simulink model "tp4_partie4"  (R2016a)
settings: Solver=VariableStepAuto  StartTime=0.0  StopTime=10.0  RelTol=1e-3
values from neighbouring files (symbols this model uses):
  K = [100;10]    [init.m]    (also in init_TP2_controle.m = [20;10]; init_tp3.m = [20 10]; matrices_init_tp4_partie3_4.m = place(A,-B,V))
  L = H/2    (= 0.072)    [matrices_init_tp4_partie3_4.m]
undefined symbols (not defined in the file or in its folder): DiscIntNeverNeededParam
libraries: simulink x2
settings Model: Creator=plarato  LastModifiedBy=plarato

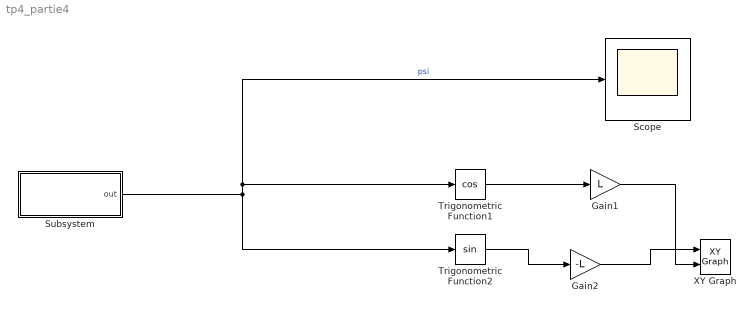
== system tp4_partie4 ==
  Gain1 : Gain  Gain=L
  Gain2 : Gain  Gain=-L
  Scope : Scope
  Subsystem : Subsystem
  Trigonometric Function1 : Trigonometry  Operator=cos
  Trigonometric Function2 : Trigonometry
  XY Graph : simulink/Sinks/XY Graph  xmin=-L  xmax=L  ymin=-L  ymax=L  st=-1
  wires:
  Trigonometric Function1/1 -> Gain1/1
  Trigonometric Function2/1 -> Gain2/1
  Gain2/1 -> XY Graph/1
  Gain1/1 -> XY Graph/2
  Subsystem/1("out ") -> Trigonometric Function2/1, Scope/1, Trigonometric Function1/1  "psi"

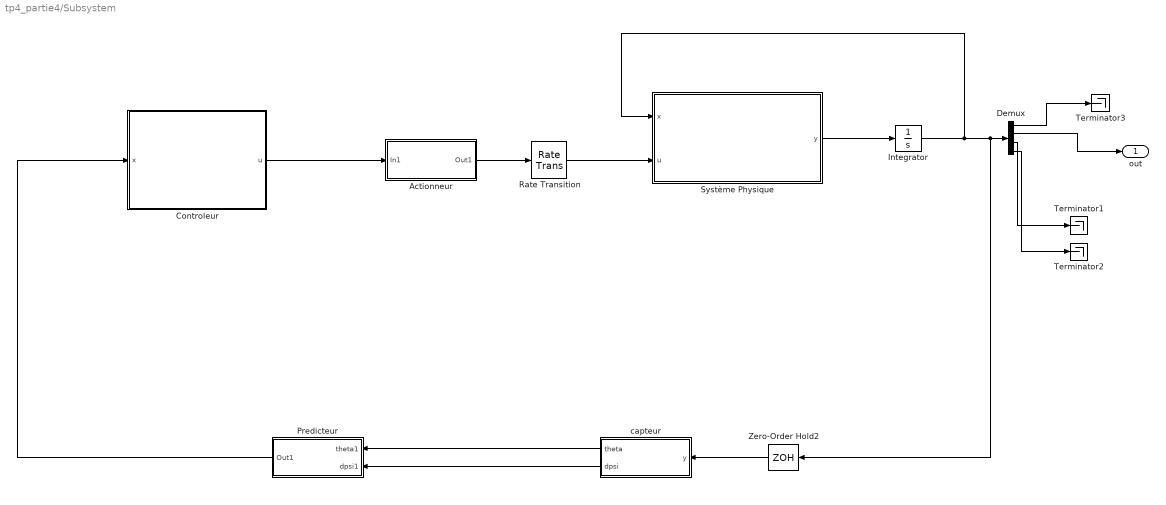
== system tp4_partie4/Subsystem ==
  Actionneur : Subsystem
  Controleur : Subsystem
  Demux : Demux
  Integrator : Integrator  InitialCondition=[pi/4 pi/3 0 0]
  Predicteur : Subsystem
  Rate Transition : RateTransition  OutPortSampleTime=0.002
  "Système Physique " : Subsystem
  Terminator1 : Terminator
  Terminator2 : Terminator
  Terminator3 : Terminator
  Zero-Order Hold2 : ZeroOrderHold  SampleTime=0.002
  "capteur " : Subsystem
  "out " : Outport
  wires:
  Controleur/1(u) -> Actionneur/1(In1)
  Actionneur/1(Out1) -> Rate Transition/1
  Integrator/1 -> "Système Physique "/1(x), Zero-Order Hold2/1, Demux/1
  Predicteur/1(Out1) -> Controleur/1(x)
  "Système Physique "/1("y ") -> Integrator/1
  Demux/3 -> Terminator1/1
  Demux/4 -> Terminator2/1
  Rate Transition/1 -> "Système Physique "/2(u)
  "capteur "/1("theta ") -> Predicteur/1(theta1)
  "capteur "/2(dpsi) -> Predicteur/2("dpsi1 ")
  Zero-Order Hold2/1 -> "capteur "/1(y)
  Demux/2 -> "out "/1
  Demux/1 -> Terminator3/1

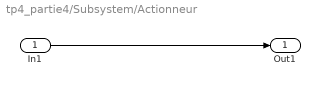
== system tp4_partie4/Subsystem/Actionneur ==
  In1 : Inport
  Out1 : Outport
  wires:
  In1/1 -> Out1/1

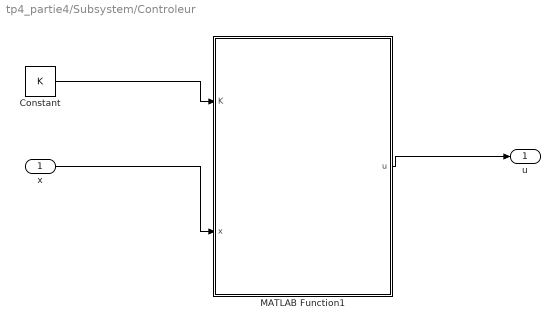
== system tp4_partie4/Subsystem/Controleur ==
  x : Inport
  Constant : Constant  Value=K
  MATLAB Function1 : MATLAB Function  TreatAsAtomicUnit=on
  u : Outport
  wires:
  MATLAB Function1/1(u) -> u/1
  x/1 -> MATLAB Function1/2(x)
  Constant/1 -> MATLAB Function1/1(K)

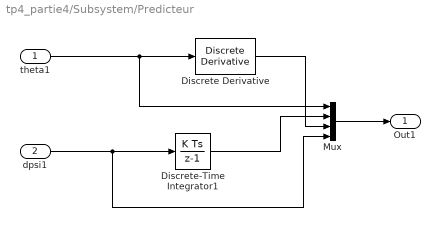
== system tp4_partie4/Subsystem/Predicteur ==
  theta1 : Inport  PortDimensions=1
  "dpsi1 " : Inport  Port=2  PortDimensions=1
  Discrete Derivative : simulink/Discrete/Discrete Derivative  gainval=1.0  ICPrevScaledInput=pi/4  OutMin=[]  OutMax=[]  OutDataType=fixdt(1, 16)  OutScaling=2^-10  DoSatur=off
  Discrete-Time Integrator1 : DiscreteIntegrator  InitialConditionSetting=State (most efficient)  SampleTime=-1  ICPrevOutput=DiscIntNeverNeededParam  ICPrevScaledInput=DiscIntNeverNeededParam
  Mux : Mux
  Out1 : Outport  PortDimensions=4
  wires:
  theta1/1 -> Mux/1, Discrete Derivative/1
  Mux/1 -> Out1/1
  Discrete-Time Integrator1/1 -> Mux/2
  "dpsi1 "/1 -> Mux/4, Discrete-Time Integrator1/1
  Discrete Derivative/1 -> Mux/3

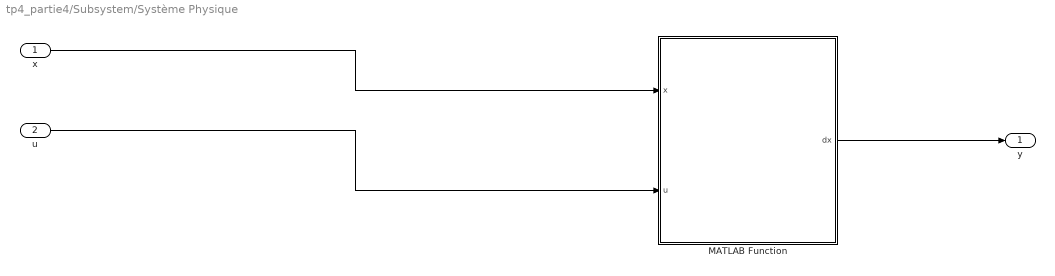
== system tp4_partie4/Subsystem/Système Physique  ==
  x : Inport
  u : Inport  Port=2
  MATLAB Function : MATLAB Function  TreatAsAtomicUnit=on
  "y " : Outport
  wires:
  MATLAB Function/1(dx) -> "y "/1
  u/1 -> MATLAB Function/2(u)
  x/1 -> MATLAB Function/1(x)

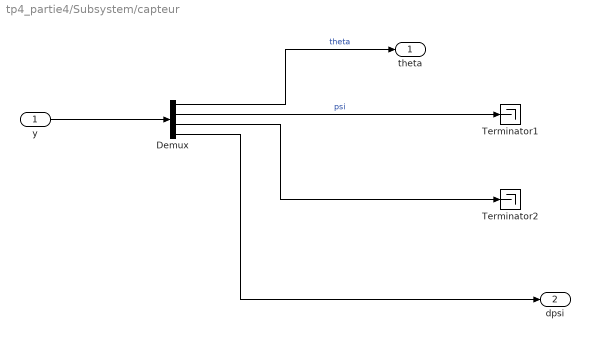
== system tp4_partie4/Subsystem/capteur  ==
  y : Inport  PortDimensions=4
  Demux : Demux
  Terminator1 : Terminator
  Terminator2 : Terminator
  "theta " : Outport  PortDimensions=1
  dpsi : Outport  Port=2  PortDimensions=1
  wires:
  Demux/1 -> "theta "/1  "theta"
  y/1 -> Demux/1
  Demux/3 -> Terminator2/1
  Demux/2 -> Terminator1/1  "psi"
  Demux/4 -> dpsi/1

== matlab function tp4_partie4/Subsystem/Controleur/MATLAB Function1 ==
  data: K input; x input; u output
%Controleur
function u = fcn(K, x)
%#codegen
ue=0;
%K=[20;10];
%K = [0.67; 19.9053; 1.0747; 1.9614];


xe = [0;0;0;0];

u = ue + K'*(x - xe);

== matlab function tp4_partie4/Subsystem/Système Physique /MATLAB Function ==
  data: x input; dx output; u input
function dx   = fonction( x, u)
%   Dynamic equations of motion of the segway on an axis.
%   Inputs: - x = [theta psi dtheta dpsi]
%               theta: average angle of the wheels      [rad]
%               psi: body pitch angle                   [rad]
%               dtheta: average velocity of the wheels  [rad/s]
%               dpsi: body pitch velocity               [rad/s]
%          - u: DC motor voltage (same value for both motors) [V]

    % State
    psi = x(2);
    dtheta = x(3);
    dpsi = x(4);

    % Parameters
    
    g = 9.81;           % gravity acceleration [m/sec^2]
    m = 0.03;           % wheel weight [kg]
    R = 0.04;           % wheel radius [m]
    Jw = m*R^2/2;       % wheel inertia moment [kg*m^2]
    M = 0.6;            % body weight [kg]
    H = 0.144;          % body height [m]
    L = H/2;            % distance of the center of mass from the wheel axle [m]
    Jpsi = M*L^2/3;     % body pitch inertia [kgm^2]
    Jm = 1e-5;          % DC motor inertia moment [kgm^2]
    Rm = 6.69;          % DC motor resistance [Ohm]
    Kb = 0.468;         % DC motor back EMF constant [Vsec/rad]
    Kt = 0.317;         % DC motor torque constant [Nm/A]
    n = 1;              % gear ratio
    fm = 0.0022;        % friction coefficient between body and DC motor
    fw = 0;             % friction coefficient between wheel and floor
    
    % Equations of motion
    c1 = (2*m+M)*R^2 + 2*Jw + 2*n^2*Jm;
    c2 = M*L*R*cos(psi) - 2*n^2*Jm;
    c3 = -M*L*R*dpsi^2*sin(psi);
    c4 = M*L^2 + Jpsi + 2*n^2*Jm;
    c5 = -M*g*L*sin(psi);

    alpha = Kt/Rm;
    beta = Kt*Kb/Rm + fm;

    Ftheta = alpha*(2*u) - 2*(beta+fw)*dtheta + 2*beta*dpsi;
    Fpsi = -alpha*(2*u) + 2*beta*dtheta - 2*beta*dpsi;

    ddtheta = (c4*c3 - c2*c5 + c4*Ftheta - c2*Fpsi)/(c4*c1 - c2^2);
    ddpsi = (Fpsi- c2*ddtheta - c5)/c4;
    dx = [dtheta dpsi ddtheta ddpsi]';

end

% Matrices of the linearized system
% E = [(2*m+M)*R^2+2*Jw+2*Jm   M*L*R-2*Jm; M*L*R-2*Jm   M*L^2+Jpsi+2*Jm];
% detE = det(E);

% alpha = Kt/Rm;
% beta = Kt*Kb/Rm + fm;

% A32 = -M*g*L*E(1,2)/detE;
% A42 = M*g*L*E(1,1)/detE;
% A33 = -(beta*E(2,2)+2*beta*E(1,2))/detE;
% A43 = (beta*E(1,2)+2*beta*E(1,1))/detE;
% A34 = beta*(E(2,2)+2*E(1,2))/detE;
% A44 = -beta*(E(1,2)+2*E(1,1))/detE;

% B3 = alpha*(E(2,2)/2+E(1,2))/detE;
% B4 = -alpha*(E(1,2)/2+E(1,1))/detE;

% A = [0 0 1 0;0 0 0 1; 0 A32 A33 A34; 0 A42 A43 A44];
% B = [0 0 2*B3 2*B4];
